simulink model "blockdemo"  (Simulink 6.3)
settings: Solver=FixedStepDiscrete  StartTime=0  StopTime=160  FixedStep=1  RelTol=1e-3
InitFcn:
  | %% DSPBuilder Start
  | alt_dspbuilder_update_model(bdroot)
  | %% DSPBuilder End
libraries: allblocks_alteradspbuilder2 x6, simulink x2
settings Model: Creator=mjervis  LastModifiedBy=delphick
settings DebuggingCC: MultiTaskDSMMsg=error

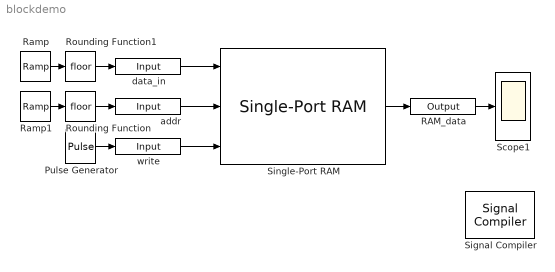
== system blockdemo ==
  Pulse Generator : DiscretePulseGenerator  Period=64  PulseWidth=32  PhaseDelay=16
      settings: AttributesFormatString=Period = %<Period>\nPulse Width = %<PulseWidth>\nPhase Delay = %<PhaseDelay>
  RAM_data : allblocks_alteradspbuilder2/Output  iofile=C:\workspace_clean\Documentation\DesignExamples\Tutorials\UnitBlocks\Storage\SinglePortRAM\tb_blockdemo\blockdemo_RAM_data.capture  BusType=Unsigned Integer  bwl=8  bwr=0  PORTTYPE=Output
  Ramp : simulink/Sources/Ramp  slope=1  start=0  X0=0
  Ramp1 : simulink/Sources/Ramp  slope=1  start=0  X0=4
  Rounding Function : Rounding
  Rounding Function1 : Rounding
  Scope1 : Scope
      settings: TimeRange=160  YMin=0  YMax=160  SampleInput=on  SampleTime=1
  Signal Compiler : allblocks_alteradspbuilder2/Signal Compiler  DeviceFamily=Cyclone III  DeviceName=AUTO  EnableSignalTap=off  SignalTapDepth=128  UseBoardBlock=off  StpUseDefaultClock=on  StpClock=clock
  Single-Port RAM : allblocks_alteradspbuilder2/Single-Port RAM  numwords=64  BusType=Inferred  bwl=8  bwr=0  memory_type=AUTO  ram_type=SingleRAM  initialization=From MATLAB array  init_file=input.hex  init_array=[63:-1:0]  register_outputs=off  use_ena=off  ClockPhase=1
      settings: AttributesFormatString=Initialization = %<init_array>\nRegister outputs = %<register_outputs>
  addr : allblocks_alteradspbuilder2/Input  iofile=C:\workspace_clean\Documentation\DesignExamples\Tutorials\UnitBlocks\Storage\SinglePortRAM\tb_blockdemo\blockdemo_addr.salt  BusType=Unsigned Integer  bwl=6  bwr=0  SpecifyClock=off  clock=default_clock  PORTTYPE=Input
  data_in : allblocks_alteradspbuilder2/Input  iofile=C:\workspace_clean\Documentation\DesignExamples\Tutorials\UnitBlocks\Storage\SinglePortRAM\tb_blockdemo\blockdemo_data_in.salt  BusType=Unsigned Integer  bwl=8  bwr=0  SpecifyClock=off  clock=default_clock  PORTTYPE=Input
  write : allblocks_alteradspbuilder2/Input  iofile=C:\workspace_clean\Documentation\DesignExamples\Tutorials\UnitBlocks\Storage\SinglePortRAM\tb_blockdemo\blockdemo_write.salt  BusType=Single Bit  bwl=3  bwr=0  SpecifyClock=off  clock=default_clock  PORTTYPE=Input
  wires:
  data_in/1 -> Single-Port RAM/1
  addr/1 -> Single-Port RAM/2
  write/1 -> Single-Port RAM/3
  Single-Port RAM/1 -> RAM_data/1
  Ramp/1 -> Rounding Function1/1
  Pulse Generator/1 -> write/1
  Ramp1/1 -> Rounding Function/1
  Rounding Function/1 -> addr/1
  RAM_data/1 -> Scope1/1
  Rounding Function1/1 -> data_in/1
